simulink model "gm_Transformation_V12"  (R2022a)
settings: Solver=FixedStepDiscrete  StartTime=0.0  StopTime=10.0  RelTol=1e-3
InitFcn:
  | Ts_xadc = 0.1;
undefined symbols (not defined in the file or in its folder): T_25MHz, T_mech
libraries: hdlsllib x14, simulink x13, hdlmdlgenlib x6, simulink_need_slupdate x1
(part 1 of 4)
settings Model: Creator=trichte  LastModifiedBy=Andre Merx
settings SolverCC: AlgebraicLoopSolver=TrustRegion
settings DataIOCC: LimitDataPoints=on  SaveFormat=Array  SaveOutput=off  SaveTime=off  ReturnWorkspaceOutputs=off
settings OptimizationCC: BlockReduction=off  ConditionallyExecuteInputs=off  DefaultParameterBehavior=Inlined  LifeSpan=inf
settings DebuggingCC: AlgebraicLoopMsg=error  SolverPrmCheckMsg=warning  InheritedTsInSrcMsg=none  SingleTaskRateTransMsg=error  UnconnectedInputMsg=warning  UnconnectedOutputMsg=warning  UnconnectedLineMsg=warning  AllowSymbolicDim=off  StrictBusMsg=ErrorOnBusTreatedAsVector  SFUnexpectedBacktrackingDiag=warning  SFNoUnconditionalDefaultTransitionDiag=warning  SFExecutionAtInitializationDiag=none  SFMachineParentedDataDiag=warning  ArithmeticOperatorsInVariantConditions=warning
settings HardwareCC: ProdBitPerPointer=32  ProdBitPerSizeT=32  ProdBitPerPtrDiffT=32  ProdLargestAtomicFloat=None  ProdIntDivRoundTo=Undefined  ProdEndianess=Unspecified  ProdWordSize=32  ProdHWDeviceType=ASIC/FPGA->ASIC/FPGA  ProdEqTarget=off
settings ModelReferenceCC: PropagateSignalLabelsOutOfModel=off
settings SFSimCC: SimUseLocalCustomCode=off  CustomCodeUndefinedFunction=UseInterfaceOnly
settings RTWCC: RTWUseLocalCustomCode=off
settings CodeAppCC: StateflowObjectComments=on
settings GRTTargetCC: TargetLangStandard=C89/C90 (ANSI)
settings ConfigComp: CovMetricSettings=dw  CovSaveCumulativeToWorkspaceVar=on  CovSaveSingleToWorkspaceVar=on  CovExternalEMLEnable=off  CovSFcnEnable=off

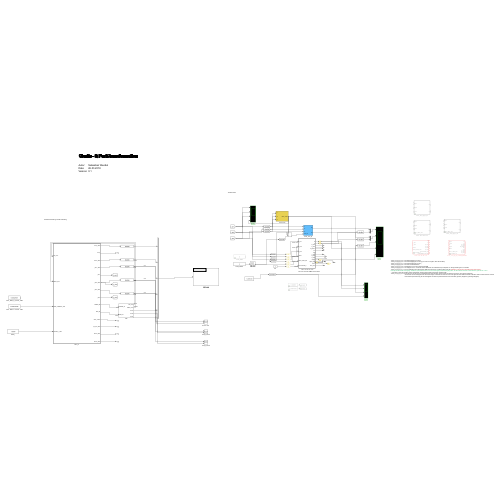
[thumbnail: Simulink's stored preview of the top-level diagram]
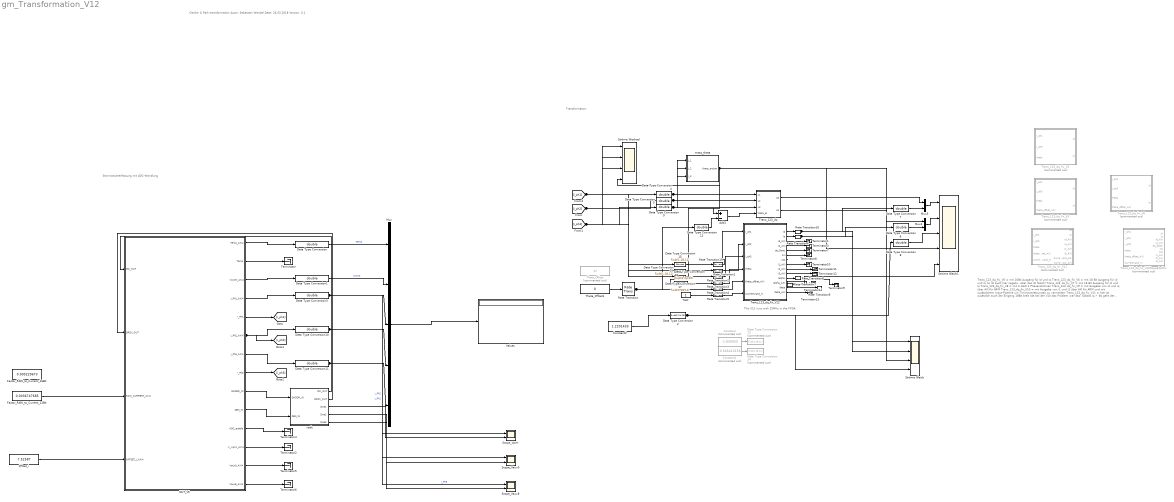
== system gm_Transformation_V12 ==
  note: Clarke- & Park-transformation
      |
      | Autor: Sebastian Wendel
      | Date: 26.03.2018
      | Version: 0.1
  note: Transformation
  note: Stromistwererfassung mit ADC-Wandlung
  note: Trans_123_dq_fix_V5 = mit 16Bit Ausgang für id und iq
      | Trans_123_dq_fix_V6 = mit 18 Bit Ausgang für id und iq (iq ist auch hier negativ, aber das ist falsch)
      | Trans_123_dq_fix_V7 = mit 18 Bit Ausgang für id und iq
      | Trans_123_dq_fix_V8 = mit 3 statt 2 Phasenströmen
      | Trans_123_dq_fix_V9 = mit Ausgabe von id und iq über AXI für ARM
      | Trans_123_dq_fix_V10 = mit Ausgabe von i1 und i3 über AXI für ARM und mit zusätzlichem Input-Pipeline um Timingverletzungen zu vermeiden
      | Trans_123_dq_fix_V11 = hier ist zusätzlich auch der Eingang 18Bit breit (da bei der V10 das Problem war das: Sobald iq > 9A geht der Trans-Block nicht mehr richtig...
      | Das liegt an den 16 Bit am Eingang. Sobald ich (wie bei den neunen V11 schon korregiert) 18 Bit am EIngang habe, ist das Problem behoben und der Bereich geht bis bis +/-36 A
      | ...ansonsten is alles wie gehabt. Wegen einheitlichen 18 Bit für alle Größem wird jedoch 18 Bit genutzt!
      | Trans_123_dq_fix_V12 = habe hier nun die dq-Trans von Saidi Said nicht mehr benutzt und bin auf die Verwendung von sinus und cosinus gewechselt.
      | da ich diese bei den VoltageVectors ohnehin benötige. Und hierdurch habe ich auch einen gleichen theta-offset für beide. Außerdem wollte ich alle 3 Ströme nehmen
      | Nach realer Implementierung ist die Genauigkeit von dieser dq-Transformation auch wesentlich genauer (doppelt so gute Bitgenauigkeit)
  note: This V12 runs with 25MHz in the FPGA.
  Add1 : Sum  Inputs=+-  OutDataTypeStr=Inherit: Same as accumulator
  Constant : Constant  Commented=on  Value=-1.839355
  Constant1 : Constant  Commented=on  Value=0.545410156
  Constant2 : Constant  Value=1.2201433
  DUT_V5 : Subsystem  TreatAsAtomicUnit=on
  Data Type Conversion{,1,3..12} (12 alike) : DataTypeConversion  OutDataTypeStr=double  SaturateOnIntegerOverflow=off  RndMeth=Floor
  Data Type Conversion13 : DataTypeConversion  Commented=on  OutDataTypeStr=fixdt(1,18,11)  SaturateOnIntegerOverflow=off  RndMeth=Floor
  Data Type Conversion14 : DataTypeConversion  Commented=on  OutDataTypeStr=fixdt(1,18,11)  SaturateOnIntegerOverflow=off  RndMeth=Floor
  Data Type Conversion15 : DataTypeConversion  OutDataTypeStr=fixdt(1,18,11)  SaturateOnIntegerOverflow=off  RndMeth=Floor
  Data Type Conversion16 : DataTypeConversion  OutDataTypeStr=fixdt(1,18,11)  SaturateOnIntegerOverflow=off  RndMeth=Floor
  Data Type Conversion17 : DataTypeConversion  OutDataTypeStr=fixdt(1,18,11)  SaturateOnIntegerOverflow=off  RndMeth=Floor
  Data Type Conversion18 : DataTypeConversion  OutDataTypeStr=fixdt(1,24,20)  SaturateOnIntegerOverflow=off  RndMeth=Floor
  Data Type Conversion2 : DataTypeConversion  OutDataTypeStr=fixdt(1,24,20)  SaturateOnIntegerOverflow=off  RndMeth=Floor
  Factor_RAW_to_Current_12Bit : Constant  Value=0.0036747685  OutDataTypeStr=fixdt(0,24,24)
  Factor_RAW_to_Current_16Bit : Constant  Value=0.000229673  OutDataTypeStr=fixdt(0,24,24)
  Mux : Mux  Inputs=5
  Mux3 : Mux  Inputs=2
  Mux4 : Mux  Inputs=2
  Offset_i : Constant  Value=7.52587  OutDataTypeStr=fixdt(0,16,11)
  Rate Transition{,6..9,16} (6 alike) : RateTransition  OutPortSampleTime=T_mech
  Rate Transition{1..5,19} (6 alike) : RateTransition  OutPortSampleTime=T_25MHz
  Scope_Vaux0 : Scope  NumInputPorts=2
  Scope_Vaux8 : Scope  NumInputPorts=2
  Scope_VpVn : Scope  NumInputPorts=2
  Ströme Gleich : Scope  NumInputPorts=4
  Ströme Gleich1 : Scope  NumInputPorts=5
  Ströme Wechsel : Scope  NumInputPorts=4
  Terminator{,1..14} (15 alike) : Terminator
  Test : Constant  OutDataTypeStr=boolean  SampleTime=T_mech
  Theta_Offset : Constant  Commented=on  Value=pi  OutDataTypeStr=fixdt(1,24,20)
  Theta_Offset1 : Constant  Value=0  OutDataTypeStr=fixdt(1,24,20)
  Trans_123_dq : Subsystem
  Trans_123_dq_fix_V11 : Subsystem  Commented=on  TreatAsAtomicUnit=on
  Trans_123_dq_fix_V12 : Subsystem  TreatAsAtomicUnit=on
  Trans_123_dq_fix_V12DoppelteMul : Subsystem  Commented=on  TreatAsAtomicUnit=on
  Trans_123_dq_fix_V3 : Subsystem  Commented=on  TreatAsAtomicUnit=on
  Trans_123_dq_fix_V5 : Subsystem  Commented=on  TreatAsAtomicUnit=on
  Trans_123_dq_fix_V6 : Subsystem  Commented=on  TreatAsAtomicUnit=on
  Values : Display
      settings: Format=hex (Stored Integer)
  meas_theta : Subsystem
  xadc : Subsystem
  wires:
  Trans_123_dq_fix_V12/12(ialpha_AXI) -> Terminator14/1
  Trans_123_dq_fix_V12/14(ibeta_AXI) -> Terminator13/1
  Trans_123_dq_fix_V12/13(ibeta) -> Rate Transition9/1
  Trans_123_dq_fix_V12/11(ialpha) -> Rate Transition8/1
  Rate Transition/1 -> Data Type Conversion12/1, Rate Transition4/1
  Data Type Conversion18/1 -> Rate Transition3/1
  Data Type Conversion17/1 -> Rate Transition2/1
  Data Type Conversion16/1 -> Rate Transition1/1
  Data Type Conversion15/1 -> Rate Transition19/1
  Trans_123_dq_fix_V12/7(cos) -> Rate Transition7/1
  Rate Transition6/1 -> Data Type Conversion6/1, Ströme Gleich/2
  Rate Transition16/1 -> Data Type Conversion7/1, Ströme Gleich/1
  Rate Transition5/1 -> Trans_123_dq_fix_V12/6(CurrentValid_in)
  Rate Transition4/1 -> Trans_123_dq_fix_V12/5(theta_offset_AXI)
  Rate Transition3/1 -> Trans_123_dq_fix_V12/4(theta)
  Rate Transition2/1 -> Trans_123_dq_fix_V12/3(i_ph3)
  Rate Transition1/1 -> Trans_123_dq_fix_V12/2(i_ph2)
  Rate Transition19/1 -> Trans_123_dq_fix_V12/1(i_ph1)
  Theta_Offset1/1 -> Rate Transition/1
  Trans_123_dq_fix_V12/10(i3_AXI) -> Terminator12/1
  Trans_123_dq_fix_V12/9(i2_AXI) -> Terminator11/1
  Constant2/1 -> Data Type Conversion2/1
  Constant1/1 -> Data Type Conversion14/1
  Constant/1 -> Data Type Conversion13/1
  Trans_123_dq_fix_V12/8(i1_AXI) -> Terminator10/1
  Test/1 -> Rate Transition5/1
  Rate Transition7/1 -> Terminator9/1, Ströme Gleich1/5
  [i_ph3] -> Data Type Conversion9/1, Data Type Conversion17/1, Ströme Wechsel/3
  [i_ph1] -> Data Type Conversion4/1, Data Type Conversion15/1, Ströme Wechsel/1
  Trans_123_dq_fix_V12/6(sin) -> Terminator8/1
  Trans_123_dq_fix_V12/5(dq_Done) -> Terminator7/1
  Trans_123_dq_fix_V12/3(id_AXI) -> Terminator1/1
  Trans_123_dq_fix_V12/4(iq_AXI) -> Terminator3/1
  Add1/1 -> Trans_123_dq/4(theta_el)
  Data Type Conversion12/1 -> Add1/2
  Trans_123_dq_fix_V12/2(iq) -> Rate Transition6/1
  Trans_123_dq_fix_V12/1(id) -> Rate Transition16/1
  [i_ph2] -> Data Type Conversion5/1, Data Type Conversion16/1, Ströme Wechsel/2
  DUT_V5/8(i_Ph3) -> [i_ph3]
  DUT_V5/5(i_Ph1) -> [i_ph1]
  Data Type Conversion5/1 -> Trans_123_dq/2(L2), meas_theta/2(I_2)
  Data Type Conversion9/1 -> Trans_123_dq/3(L3), meas_theta/3(I_3)
  Data Type Conversion4/1 -> Trans_123_dq/1(L1), meas_theta/1(I_1)
  meas_theta/1(theta_arctan) -> Add1/1, Data Type Conversion18/1, Ströme Gleich1/4, Ströme Gleich/3, Ströme Wechsel/4
  Data Type Conversion8/1 -> Ströme Gleich1/3
  Mux4/1 -> Ströme Gleich1/2
  Data Type Conversion6/1 -> Mux4/2
  Data Type Conversion7/1 -> Mux3/2
  Mux3/1 -> Ströme Gleich1/1
  Trans_123_dq/2(Uq) -> Mux4/1
  Trans_123_dq/1(Ud) -> Mux3/1
  Data Type Conversion2/1 -> Data Type Conversion8/1, Ströme Gleich/4
  xadc/5(Sine3) -> Scope_Vaux8/2
  xadc/4(Sine2) -> Scope_Vaux0/2
  xadc/3(Sine1) -> Scope_VpVn/2
  DUT_V5/14(Vaux8_AXI4) -> Terminator6/1
  DUT_V5/13(Vaux0_AXI4) -> Terminator5/1
  DUT_V5/12(V_VpVn_AXI4) -> Terminator2/1
  Offset_i/1 -> DUT_V5/4(OFFSET_I_AXI4)
  Factor_RAW_to_Current_12Bit/1 -> DUT_V5/3(RAW_CURRENT_AXI4)
  DUT_V5/11(ADC_enable) -> Terminator4/1
  DUT_V5/2(Temp) -> Terminator/1
  xadc/1(DO_OUT) -> DUT_V5/1(DO_OUT)
  xadc/2(DRDY_OUT) -> DUT_V5/2(DRDY_OUT)
  DUT_V5/10(DEN_IN) -> xadc/2(DEN_IN)
  DUT_V5/9(DADDR_IN) -> xadc/1(DADDR_IN)
  Data Type Conversion1/1 -> Mux/2  "VccInt"
  Data Type Conversion11/1 -> Mux/5, Scope_Vaux8/1  "i_Ph3"
  Data Type Conversion10/1 -> Mux/4, Scope_Vaux0/1  "i_Ph2"
  Data Type Conversion3/1 -> Mux/3, Scope_VpVn/1  "i_Ph1"
  Data Type Conversion/1 -> Mux/1  "Temp"
  Mux/1 -> Values/1
  DUT_V5/6(i_Ph2_AXI4) -> Data Type Conversion10/1, [i_ph2]
  DUT_V5/7(i_Ph3_AXI4) -> Data Type Conversion11/1
  DUT_V5/4(i_Ph1_AXI4) -> Data Type Conversion3/1
  DUT_V5/3(VccInt_AXI4) -> Data Type Conversion1/1
  DUT_V5/1(Temp_AXI4) -> Data Type Conversion/1

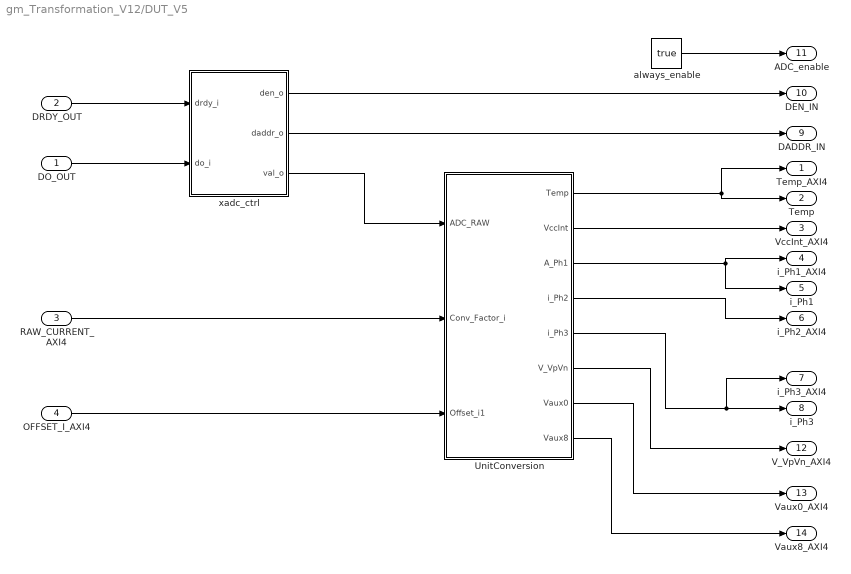
== system gm_Transformation_V12/DUT_V5 ==
  DO_OUT : Inport
  DRDY_OUT : Inport  Port=2
  RAW_CURRENT_AXI4 : Inport  Port=3
  OFFSET_I_AXI4 : Inport  Port=4
  UnitConversion : Subsystem
  always_enable : Constant  Value=true  OutDataTypeStr=boolean
  xadc_ctrl : MATLAB Function  TreatAsAtomicUnit=on
  Temp_AXI4 : Outport  VectorParamsAs1DForOutWhenUnconnected=off
  Temp : Outport  Port=2  VectorParamsAs1DForOutWhenUnconnected=off
  VccInt_AXI4 : Outport  Port=3  VectorParamsAs1DForOutWhenUnconnected=off
  i_Ph1_AXI4 : Outport  Port=4  VectorParamsAs1DForOutWhenUnconnected=off
  i_Ph1 : Outport  Port=5  VectorParamsAs1DForOutWhenUnconnected=off
  i_Ph2_AXI4 : Outport  Port=6  VectorParamsAs1DForOutWhenUnconnected=off
  i_Ph3_AXI4 : Outport  Port=7  VectorParamsAs1DForOutWhenUnconnected=off
  i_Ph3 : Outport  Port=8  VectorParamsAs1DForOutWhenUnconnected=off
  DADDR_IN : Outport  Port=9  VectorParamsAs1DForOutWhenUnconnected=off
  DEN_IN : Outport  Port=10  VectorParamsAs1DForOutWhenUnconnected=off
  ADC_enable : Outport  Port=11  VectorParamsAs1DForOutWhenUnconnected=off
  V_VpVn_AXI4 : Outport  Port=12  VectorParamsAs1DForOutWhenUnconnected=off
  Vaux0_AXI4 : Outport  Port=13  VectorParamsAs1DForOutWhenUnconnected=off
  Vaux8_AXI4 : Outport  Port=14  VectorParamsAs1DForOutWhenUnconnected=off
  wires:
  UnitConversion/8(Vaux8) -> Vaux8_AXI4/1
  UnitConversion/7(Vaux0) -> Vaux0_AXI4/1
  OFFSET_I_AXI4/1 -> UnitConversion/3(Offset_i1)
  UnitConversion/6(V_VpVn) -> V_VpVn_AXI4/1
  RAW_CURRENT_AXI4/1 -> UnitConversion/2(Conv_Factor_i)
  always_enable/1 -> ADC_enable/1
  xadc_ctrl/2(daddr_o) -> DADDR_IN/1
  xadc_ctrl/1(den_o) -> DEN_IN/1
  DO_OUT/1 -> xadc_ctrl/2(do_i)
  DRDY_OUT/1 -> xadc_ctrl/1(drdy_i)
  UnitConversion/1(Temp) -> Temp_AXI4/1, Temp/1
  UnitConversion/2(VccInt) -> VccInt_AXI4/1
  UnitConversion/4(i_Ph2) -> i_Ph2_AXI4/1
  UnitConversion/3(A_Ph1) -> i_Ph1_AXI4/1, i_Ph1/1
  UnitConversion/5(i_Ph3) -> i_Ph3_AXI4/1, i_Ph3/1
  xadc_ctrl/3(val_o) -> UnitConversion/1(ADC_RAW)

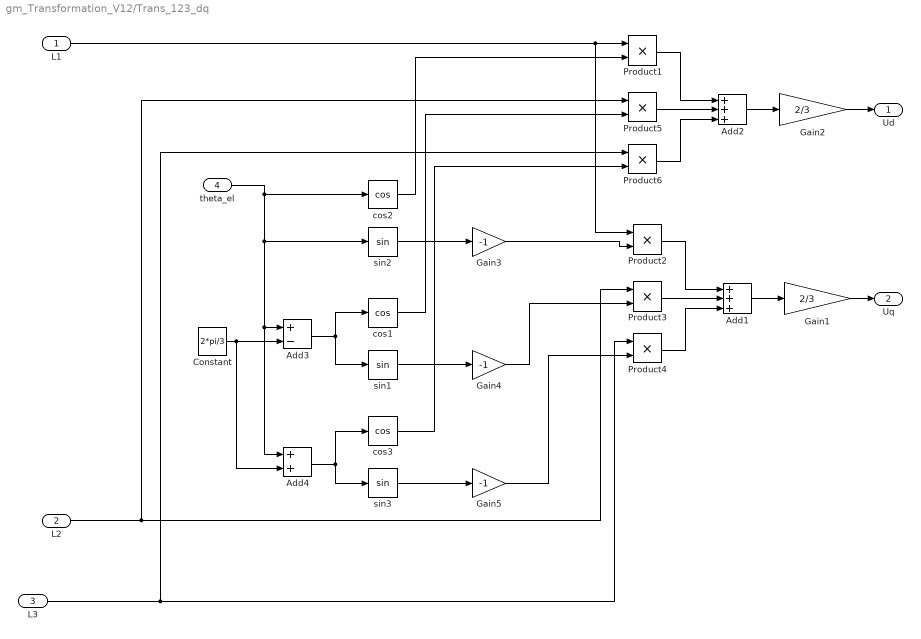
== system gm_Transformation_V12/Trans_123_dq ==
  L1 : Inport
  L2 : Inport  Port=2
  L3 : Inport  Port=3
  theta_el : Inport  Port=4
  Add1 : Sum  Inputs=+++
  Add2 : Sum  Inputs=+++
  Add3 : Sum  Inputs=+-
  Add4 : Sum
  Constant : Constant  Value=2*pi/3  SampleTime=T_mech
  Gain1 : Gain  Gain=2/3
  Gain2 : Gain  Gain=2/3
  Gain3 : Gain  Gain=-1
  Gain4 : Gain  Gain=-1
  Gain5 : Gain  Gain=-1
  Product{1..6} (6 alike) : Product  RndMeth=Zero
  cos1 : Trigonometry  Operator=cos
  cos2 : Trigonometry  Operator=cos
  cos3 : Trigonometry  Operator=cos
  sin1 : Trigonometry
  sin2 : Trigonometry
  sin3 : Trigonometry
  Ud : Outport  VectorParamsAs1DForOutWhenUnconnected=off
  Uq : Outport  Port=2  VectorParamsAs1DForOutWhenUnconnected=off
  wires:
  cos2/1 -> Product1/2
  cos1/1 -> Product5/2
  cos3/1 -> Product6/2
  Product1/1 -> Add2/1
  Add4/1 -> sin3/1, cos3/1
  Add3/1 -> sin1/1, cos1/1
  Constant/1 -> Add4/2, Add3/2
  theta_el/1 -> sin2/1, Add4/1, Add3/1, cos2/1
  Product3/1 -> Add1/2
  Product2/1 -> Add1/1
  Add1/1 -> Gain1/1
  Product4/1 -> Add1/3
  Product5/1 -> Add2/2
  Add2/1 -> Gain2/1
  Product6/1 -> Add2/3
  Gain2/1 -> Ud/1
  Gain1/1 -> Uq/1
  L1/1 -> Product1/1, Product2/1
  L2/1 -> Product5/1, Product3/1
  L3/1 -> Product6/1, Product4/1
  sin2/1 -> Gain3/1
  sin1/1 -> Gain4/1
  sin3/1 -> Gain5/1
  Gain3/1 -> Product2/2
  Gain4/1 -> Product3/2
  Gain5/1 -> Product4/2

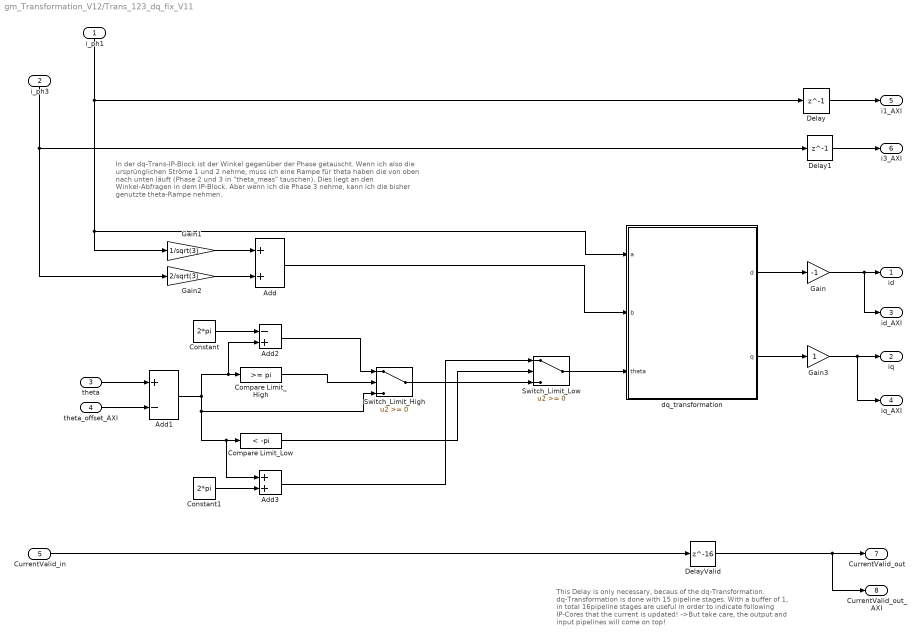
== system gm_Transformation_V12/Trans_123_dq_fix_V11 ==
  note: In der dq-Trans-IP-Block ist der Winkel gegenüber der Phase getauscht.
      | Wenn ich also die ursprünglichen Ströme 1 und 2 nehme,
      |  muss ich eine Rampe für theta haben die von oben nach unten läuft
      | (Phase 2 und 3 in "theta_meas" tauschen).
      | Dies liegt an den Winkel-Abfragen in dem IP-Block.
      | Aber wenn ich die Phase 3 nehme, kann ich die bisher genutzte theta-Rampe nehmen.
  note: This Delay is only necessary, becaus of the dq-Transformation.
      | dq-Transformation is done with 15 pipeline stages.
      | With a buffer of 1, in total 16pipeline stages are useful in order to
      |  indicate following IP-Cores that the current is updated!
      | ->But take care, the output and input pipelines will come on top!
  i_ph1 : Inport
  i_ph3 : Inport  Port=2
  theta : Inport  Port=3
  theta_offset_AXI : Inport  Port=4
  CurrentValid_in : Inport  Port=5
  Add : Sum
  Add1 : Sum  Inputs=+-  OutDataTypeStr=Inherit: Same as accumulator
  Add2 : Sum  Inputs=-+  OutDataTypeStr=Inherit: Same as first input
  Add3 : Sum  OutDataTypeStr=Inherit: Same as first input
  Compare Limit_High : simulink/Logic and Bit Operations/Compare To Constant  relop=>=  const=pi  OutDataTypeStr=boolean
  Compare Limit_Low : simulink/Logic and Bit Operations/Compare To Constant  relop=<  const=-pi  OutDataTypeStr=boolean
  Constant : Constant  Value=2*pi  OutDataTypeStr=fixdt(1,24,20)  SampleTime=-1
  Constant1 : Constant  Value=2*pi  OutDataTypeStr=fixdt(1,24,20)  SampleTime=-1
  Delay : Delay  DelayLength=1
  Delay1 : Delay  DelayLength=1
  DelayValid : Delay  DelayLength=16
  Gain : Gain  Gain=-1  OutDataTypeStr=fixdt(1,18,11)
  Gain1 : Gain  Gain=1/sqrt(3)  OutDataTypeStr=Inherit: Same as input
  Gain2 : Gain  Gain=2/sqrt(3)  OutDataTypeStr=Inherit: Same as input
  Gain3 : Gain  OutDataTypeStr=fixdt(1,18,11)
  Switch_Limit_High : Switch  OutDataTypeStr=fixdt(1,24,20)  SaturateOnIntegerOverflow=off  InputSameDT=off
  Switch_Limit_Low : Switch  OutDataTypeStr=fixdt(1,24,20)  SaturateOnIntegerOverflow=off  InputSameDT=off
  dq_transformation : MATLAB Function  TreatAsAtomicUnit=on
  id : Outport  VectorParamsAs1DForOutWhenUnconnected=off
  iq : Outport  Port=2  VectorParamsAs1DForOutWhenUnconnected=off
  id_AXI : Outport  Port=3  VectorParamsAs1DForOutWhenUnconnected=off
  iq_AXI : Outport  Port=4  VectorParamsAs1DForOutWhenUnconnected=off
  i1_AXI : Outport  Port=5  VectorParamsAs1DForOutWhenUnconnected=off
  i3_AXI : Outport  Port=6  VectorParamsAs1DForOutWhenUnconnected=off
  CurrentValid_out : Outport  Port=7  VectorParamsAs1DForOutWhenUnconnected=off
  CurrentValid_out_AXI : Outport  Port=8  VectorParamsAs1DForOutWhenUnconnected=off
  wires:
  CurrentValid_in/1 -> DelayValid/1
  DelayValid/1 -> CurrentValid_out/1, CurrentValid_out_AXI/1
  i_ph1/1 -> Delay/1, dq_transformation/1(a), Gain1/1
  i_ph3/1 -> Delay1/1, Gain2/1
  Delay1/1 -> i3_AXI/1
  Delay/1 -> i1_AXI/1
  Gain/1 -> id/1, id_AXI/1
  Gain3/1 -> iq/1, iq_AXI/1
  Add3/1 -> Switch_Limit_Low/1
  Constant1/1 -> Add3/2
  Add2/1 -> Switch_Limit_High/1
  Constant/1 -> Add2/1
  Compare Limit_Low/1 -> Switch_Limit_Low/2
  Compare Limit_High/1 -> Switch_Limit_High/2
  Switch_Limit_High/1 -> Switch_Limit_Low/3
  Switch_Limit_Low/1 -> dq_transformation/3(theta)
  theta_offset_AXI/1 -> Add1/2
  Add1/1 -> Compare Limit_High/1, Add2/2, Compare Limit_Low/1, Add3/1, Switch_Limit_High/3
  theta/1 -> Add1/1
  dq_transformation/1(d) -> Gain/1
  dq_transformation/2(q) -> Gain3/1
  Gain2/1 -> Add/2
  Gain1/1 -> Add/1
  Add/1 -> dq_transformation/2(b)

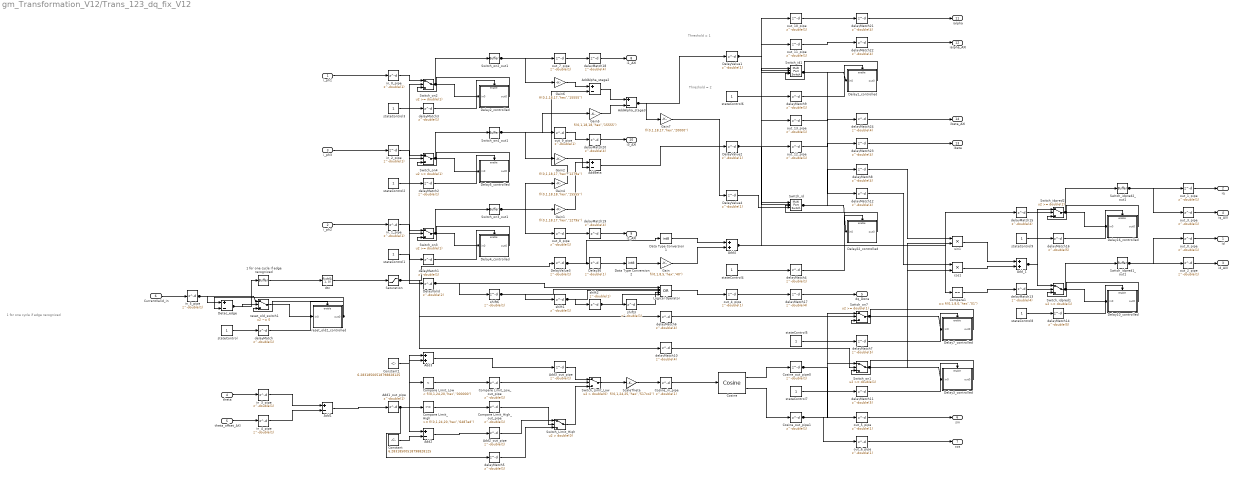
== system gm_Transformation_V12/Trans_123_dq_fix_V12 ==
  note: Threshold = 2
  note: Threshold = 1
  note: 1 for one cycle if edge recognized
  i_ph1 : Inport  OutDataTypeStr=fixdt(1, 18, 11)  PortDimensions=1  SampleTime=4e-08
  i_ph2 : Inport  Port=2  OutDataTypeStr=fixdt(1, 18, 11)  PortDimensions=1  SampleTime=4e-08
  i_ph3 : Inport  Port=3  OutDataTypeStr=fixdt(1, 18, 11)  PortDimensions=1  SampleTime=4e-08
  theta : Inport  Port=4  OutDataTypeStr=fixdt(1, 24, 20)  PortDimensions=1  SampleTime=4e-08
  theta_offset_AXI : Inport  Port=5  OutDataTypeStr=fixdt(1, 24, 20)  PortDimensions=1  SampleTime=4e-08
  CurrentValid_in : Inport  Port=6  OutDataTypeStr=boolean  PortDimensions=1  SampleTime=4e-08
  1 for one cycle if edge recognized : hdlmdlgenlib/Buffer
      settings: SourceProductBaseCode=SL
  Add1 : Sum  Inputs=+-  AccumDataTypeStr=fixdt(1, 24, 20)  OutDataTypeStr=fixdt(1, 24, 20)  SampleTime=4e-08
  Add1_out_pipe : Delay  DelayLength=double(1)  InitialCondition=0  SampleTime=4e-08
  Add2 : Sum  Inputs=+-  AccumDataTypeStr=fixdt(1, 24, 20)  OutDataTypeStr=fixdt(1, 24, 20)  SampleTime=4e-08
  Add2_out_pipe : Delay  DelayLength=double(1)  InitialCondition=0  SampleTime=4e-08
  Add3 : Sum  AccumDataTypeStr=fixdt(1, 24, 20)  OutDataTypeStr=fixdt(1, 24, 20)  SampleTime=4e-08
  Add3_out_pipe : Delay  DelayLength=double(1)  InitialCondition=0  SampleTime=4e-08
  Add4 : Sum  AccumDataTypeStr=int8  OutDataTypeStr=int8  RndMeth=Simplest  SampleTime=4e-08
  AddAlpha_stage2 : Sum  Inputs=+-  AccumDataTypeStr=fixdt(1, 18, 11)  OutDataTypeStr=fixdt(1, 18, 11)  SampleTime=4e-08
  AddAlpha_stage3 : Sum  Inputs=+-  AccumDataTypeStr=fixdt(1, 18, 11)  OutDataTypeStr=fixdt(1, 18, 11)  SampleTime=4e-08
  AddBeta : Sum  Inputs=+-  AccumDataTypeStr=fixdt(1, 18, 11)  OutDataTypeStr=fixdt(1, 18, 11)  SampleTime=4e-08
  Add_1 : Sum  AccumDataTypeStr=fixdt(1, 18, 11)  OutDataTypeStr=fixdt(1, 18, 11)  SampleTime=4e-08
  Compare Limit_High : simulink/Logic and Bit Operations/Compare To Constant  relop=>=  const="fi(0,1,24,20,\"hex\",\"6487ed\")"  OutDataTypeStr=boolean
  Compare Limit_High_out_pipe : Delay  DelayLength=double(1)  InitialCondition=0  SampleTime=4e-08
  Compare Limit_Low : simulink/Logic and Bit Operations/Compare To Constant  relop=<  const="fi(0,1,24,20,\"hex\",\"000000\")"  OutDataTypeStr=boolean
  Compare Limit_Low_out_pipe : Delay  DelayLength=double(1)  InitialCondition=0  SampleTime=4e-08
  Compare1 : simulink/Logic and Bit Operations/Compare To Constant  relop===  const="fi(0,1,8,0,\"hex\",\"01\")"  OutDataTypeStr=boolean
  Constant : Constant  Value=6.28318500518798828125  OutDataTypeStr=fixdt(1, 24, 20)  SampleTime=4e-08
  Constant1 : Constant  Value=6.28318500518798828125  OutDataTypeStr=fixdt(1, 24, 20)  SampleTime=4e-08
  Cosine : simulink/Lookup Tables/Cosine  Formula=sin(2*pi*u) and cos(2*pi*u)  NumDataPoints=(2^9)+1  OutputWordLength=16  InternalRulePriority=Precision
      settings: SourceProductBaseCode=SL
  Cosine_in_pipe : Delay  DelayLength=double(1)  InitialCondition=0  SampleTime=4e-08
  Cosine_out_pipe0 : Delay  DelayLength=double(1)  InitialCondition=0  SampleTime=4e-08
  Cosine_out_pipe1 : Delay  DelayLength=double(1)  InitialCondition=0  SampleTime=4e-08
  Data Type Conversion1 : DataTypeConversion  OutDataTypeStr=int8  SampleTime=4e-08  SaturateOnIntegerOverflow=off  RndMeth=Floor
  Data Type Conversion2 : DataTypeConversion  OutDataTypeStr=int8  SampleTime=4e-08  SaturateOnIntegerOverflow=off  RndMeth=Floor
  Delay10_controlled : Subsystem
  Delay16_controlled : Subsystem
  Delay1_controlled : Subsystem
  Delay22_controlled : Subsystem
  Delay2_controlled : Subsystem
  Delay36 : Delay  DelayLength=double(1)  InitialCondition=0  SampleTime=4e-08
  Delay3_controlled : Subsystem
  Delay4_controlled : Subsystem
  Delay5_controlled : Subsystem
  Delay7_controlled : Subsystem
  DelayValid : Delay  DelayLength=double(2)  InitialCondition=0  SampleTime=4e-08
  DelayValue{1..4} (4 alike) : Delay  DelayLength=double(1)  InitialCondition=0  SampleTime=4e-08
  Detec_edge : Sum  Inputs=+-  AccumDataTypeStr=int8  OutDataTypeStr=int8  SampleTime=4e-08
  Gain : Gain  Gain="fi(0,1,8,5,\"hex\",\"40\")"  ParamDataTypeStr=fixdt(1, 8, 5)  OutDataTypeStr=fixdt(1, 16, 5)  RndMeth=Simplest  SampleTime=4e-08
  Gain1 : Gain  Gain="fi(0,1,18,17,\"hex\",\"1279a\")"  ParamDataTypeStr=fixdt(1, 18, 17)  OutDataTypeStr=fixdt(1, 18, 11)  SampleTime=4e-08
  Gain2 : Gain  Gain="fi(0,1,18,17,\"hex\",\"1279a\")"  ParamDataTypeStr=fixdt(1, 18, 17)  OutDataTypeStr=fixdt(1, 18, 11)  SampleTime=4e-08
  Gain4 : Gain  Gain="fi(0,1,18,18,\"hex\",\"15555\")"  ParamDataTypeStr=fixdt(1, 18, 18)  OutDataTypeStr=fixdt(1, 18, 11)  SampleTime=4e-08
  Gain5 : Gain  Gain="fi(0,1,18,18,\"hex\",\"15555\")"  ParamDataTypeStr=fixdt(1, 18, 18)  OutDataTypeStr=fixdt(1, 18, 11)  SampleTime=4e-08
  Gain6 : Gain  Gain="fi(0,1,18,17,\"hex\",\"15555\")"  ParamDataTypeStr=fixdt(1, 18, 17)  OutDataTypeStr=fixdt(1, 18, 11)  SampleTime=4e-08
  Gain7 : Gain  Gain="fi(0,1,18,17,\"hex\",\"20000\")"  ParamDataTypeStr=fixdt(1, 18, 17)  OutDataTypeStr=fixdt(1, 18, 11)  SampleTime=4e-08
  Logical Operator : Logic  Operator=OR  Inputs=5  AllPortsSameDT=off  OutDataTypeStr=boolean  SampleTime=4e-08
  Saturation : Saturate  UpperLimit="fi(0,0,1,0,\"hex\",\"1\")"  LowerLimit="fi(0,0,1,0,\"hex\",\"0\")"  SampleTime=4e-08  OutDataTypeStr=fixdt(0, 1, 0)
  ScaleTheta : Gain  Gain="fi(0,1,24,25,\"hex\",\"517cc2\")"  ParamDataTypeStr=fixdt(1, 24, 25)  OutDataTypeStr=fixdt(1, 24, 20)  SampleTime=4e-08
  Switch_Limit_High : Switch  Criteria=u2 > Threshold  Threshold=double(0)  OutDataTypeStr=fixdt(1, 24, 20)  SampleTime=4e-08  SaturateOnIntegerOverflow=off  InputSameDT=off
  Switch_Limit_Low : Switch  Criteria=u2 > Threshold  Threshold=double(0)  OutDataTypeStr=fixdt(1, 24, 20)  SampleTime=4e-08  SaturateOnIntegerOverflow=off  InputSameDT=off
  Switch_id : MultiPortSwitch  Inputs=2  DataPortForDefault=Additional data port  DiagnosticForDefault=None  OutDataTypeStr=fixdt(1, 18, 11)  RndMeth=Simplest  SampleTime=4e-08  SaturateOnIntegerOverflow=off  InputSameDT=off
  Switch_id1 : MultiPortSwitch  Inputs=2  DataPortForDefault=Additional data port  DiagnosticForDefault=None  OutDataTypeStr=fixdt(1, 18, 11)  RndMeth=Simplest  SampleTime=4e-08  SaturateOnIntegerOverflow=off  InputSameDT=off
  Switch_idpred1 : Switch  Threshold=double(1)  OutDataTypeStr=fixdt(1, 18, 11)  RndMeth=Simplest  SampleTime=4e-08  SaturateOnIntegerOverflow=off  InputSameDT=off
  Switch_idpred1_out1 : hdlmdlgenlib/Buffer
      settings: SourceProductBaseCode=SL
  Switch_idpred2 : Switch  Threshold=double(2)  OutDataTypeStr=fixdt(1, 18, 11)  RndMeth=Simplest  SampleTime=4e-08  SaturateOnIntegerOverflow=off  InputSameDT=off
  Switch_idpred2_out1 : hdlmdlgenlib/Buffer
      settings: SourceProductBaseCode=SL
  Switch_on1 : Switch  Threshold=double(1)  OutDataTypeStr=fixdt(1, 16, 14)  SampleTime=4e-08  SaturateOnIntegerOverflow=off  InputSameDT=off
  Switch_on2 : Switch  Threshold=double(1)  OutDataTypeStr=fixdt(1, 18, 11)  RndMeth=Simplest  SampleTime=4e-08  SaturateOnIntegerOverflow=off  InputSameDT=off
  Switch_on2_out1 : hdlmdlgenlib/Buffer
      settings: SourceProductBaseCode=SL
  Switch_on3 : Switch  Threshold=double(1)  OutDataTypeStr=fixdt(1, 18, 11)  RndMeth=Simplest  SampleTime=4e-08  SaturateOnIntegerOverflow=off  InputSameDT=off
  Switch_on3_out1 : hdlmdlgenlib/Buffer
      settings: SourceProductBaseCode=SL
  Switch_on4 : Switch  Threshold=double(1)  OutDataTypeStr=fixdt(1, 18, 11)  RndMeth=Simplest  SampleTime=4e-08  SaturateOnIntegerOverflow=off  InputSameDT=off
  Switch_on4_out1 : hdlmdlgenlib/Buffer
      settings: SourceProductBaseCode=SL
  Switch_on7 : Switch  Threshold=double(1)  OutDataTypeStr=fixdt(1, 16, 14)  SampleTime=4e-08  SaturateOnIntegerOverflow=off  InputSameDT=off
  cos1 : Product  Inputs=**  OutDataTypeStr=fixdt(1, 18, 11)  RndMeth=Simplest  SampleTime=4e-08
  delayMatch{,1..5,9} (7 alike) : Delay  DelayLength=double(1)  InitialCondition=0  SampleTime=4e-08
  delayMatch{6,8,10,12..13,15,17..24} (14 alike) : Delay  DelayLength=double(4)  InitialCondition=0  SampleTime=4e-08
  delayMatch{7,11,14,16} (4 alike) : Delay  DelayLength=double(5)  InitialCondition=0  SampleTime=4e-08
  dtc : DataTypeConversion  OutDataTypeStr=fixdt(0, 1, 0)  SampleTime=4e-08  RndMeth=Floor
  in_0_pipe : Delay  DelayLength=double(1)  InitialCondition=0  SampleTime=4e-08
  in_1_pipe : Delay  DelayLength=double(1)  InitialCondition=0  SampleTime=4e-08
  in_2_pipe : Delay  DelayLength=double(1)  InitialCondition=0  SampleTime=4e-08
  in_3_pipe : Delay  DelayLength=double(1)  InitialCondition=0  SampleTime=4e-08
  in_4_pipe : Delay  DelayLength=double(1)  InitialCondition=0  SampleTime=4e-08
  in_5_pipe : Delay  DelayLength=double(1)  InitialCondition=0  SampleTime=4e-08
  out_0_pipe : Delay  DelayLength=double(1)  InitialCondition=0  SampleTime=4e-08
  out_10_pipe : Delay  DelayLength=double(1)  InitialCondition=0  SampleTime=4e-08
  out_11_pipe : Delay  DelayLength=double(1)  InitialCondition=0  SampleTime=4e-08
  out_12_pipe : Delay  DelayLength=double(1)  InitialCondition=0  SampleTime=4e-08
  out_13_pipe : Delay  DelayLength=double(1)  InitialCondition=0  SampleTime=4e-08
  out_1_pipe : Delay  DelayLength=double(1)  InitialCondition=0  SampleTime=4e-08
  out_2_pipe : Delay  DelayLength=double(1)  InitialCondition=0  SampleTime=4e-08
  out_3_pipe : Delay  DelayLength=double(1)  InitialCondition=0  SampleTime=4e-08
  out_4_pipe : Delay  DelayLength=double(1)  InitialCondition=0  SampleTime=4e-08
  out_5_pipe : Delay  DelayLength=double(1)  InitialCondition=0  SampleTime=4e-08
  out_6_pipe : Delay  DelayLength=double(1)  InitialCondition=0  SampleTime=4e-08
  out_7_pipe : Delay  DelayLength=double(1)  InitialCondition=0  SampleTime=4e-08
  out_8_pipe : Delay  DelayLength=double(1)  InitialCondition=0  SampleTime=4e-08
  out_9_pipe : Delay  DelayLength=double(1)  InitialCondition=0  SampleTime=4e-08
  reset_old2_controlled : Subsystem
  reset_old_switch1 : Switch  Criteria=u2 ~= 0  Threshold=double(0)  OutDataTypeStr=boolean  SampleTime=4e-08  SaturateOnIntegerOverflow=off  InputSameDT=off
  shift{1..3,6} (4 alike) : Delay  DelayLength=double(1)  InitialCondition=0  SampleTime=4e-08
  sin1 : Product  Inputs=**  OutDataTypeStr=fixdt(1, 18, 11)  RndMeth=Simplest  SampleTime=4e-08
  stateControl{,1..9} (10 alike) : Constant  OutDataTypeStr=boolean  SampleTime=4e-08
  id : Outport  SampleTime=4e-08  VectorParamsAs1DForOutWhenUnconnected=off
  iq : Outport  Port=2  SampleTime=4e-08  VectorParamsAs1DForOutWhenUnconnected=off
  id_AXI : Outport  Port=3  SampleTime=4e-08  VectorParamsAs1DForOutWhenUnconnected=off
  iq_AXI : Outport  Port=4  SampleTime=4e-08  VectorParamsAs1DForOutWhenUnconnected=off
  dq_Done : Outport  Port=5  SampleTime=4e-08  VectorParamsAs1DForOutWhenUnconnected=off
  sin : Outport  Port=6  SampleTime=4e-08  VectorParamsAs1DForOutWhenUnconnected=off
  cos : Outport  Port=7  SampleTime=4e-08  VectorParamsAs1DForOutWhenUnconnected=off
  i1_AXI : Outport  Port=8  SampleTime=4e-08  VectorParamsAs1DForOutWhenUnconnected=off
  i2_AXI : Outport  Port=9  SampleTime=4e-08  VectorParamsAs1DForOutWhenUnconnected=off
  i3_AXI : Outport  Port=10  SampleTime=4e-08  VectorParamsAs1DForOutWhenUnconnected=off
  ialpha : Outport  Port=11  SampleTime=4e-08  VectorParamsAs1DForOutWhenUnconnected=off
  ialpha_AXI : Outport  Port=12  SampleTime=4e-08  VectorParamsAs1DForOutWhenUnconnected=off
  ibeta : Outport  Port=13  SampleTime=4e-08  VectorParamsAs1DForOutWhenUnconnected=off
  ibeta_AXI : Outport  Port=14  SampleTime=4e-08  VectorParamsAs1DForOutWhenUnconnected=off
  wires:
  in_0_pipe/1 -> Switch_on2/1
  in_1_pipe/1 -> Switch_on3/1
  in_2_pipe/1 -> Switch_on4/1
  in_3_pipe/1 -> Add1/1
  in_4_pipe/1 -> Add1/2
  in_5_pipe/1 -> reset_old_switch1/1, Detec_edge/1
  delayMatch5/1 -> Switch_Limit_High/3
  Add2_out_pipe/1 -> Switch_Limit_High/1
  Add3_out_pipe/1 -> Switch_Limit_Low/1
  delayMatch15/1 -> Switch_idpred2/2
  AddAlpha_stage3/1 -> Gain7/1, DelayValue1/1
  AddBeta/1 -> DelayValue2/1
  Add_1/1 -> Switch_idpred1/1, Switch_idpred2/1
  Compare Limit_High_out_pipe/1 -> Switch_Limit_High/2
  Compare Limit_Low_out_pipe/1 -> Switch_Limit_Low/2
  delayMatch13/1 -> Switch_idpred1/2
  Constant/1 -> Add2/2
  Constant1/1 -> Add3/2
  Cosine_out_pipe0/1 -> out_5_pipe/1, Switch_on7/1
  Cosine_out_pipe1/1 -> out_6_pipe/1, Switch_on1/1
  Data Type Conversion1/1 -> Add4/1
  Data Type Conversion2/1 -> Gain/1
  Delay36/1 -> Data Type Conversion2/1
  DelayValid/1 -> Logical Operator/1, shift6/1
  DelayValue1/1 -> out_11_pipe/1, out_10_pipe/1, Switch_id1/2
  DelayValue2/1 -> out_13_pipe/1, out_12_pipe/1, Switch_id/2, Switch_id1/3
  DelayValue3/1 -> Data Type Conversion1/1, Delay36/1
  DelayValue4/1 -> Switch_id/3
  1 for one cycle if edge recognized/1 -> dtc/1
  Gain/1 -> Add4/2
  Gain1/1 -> AddBeta/1
  Gain2/1 -> AddBeta/2
  Gain4/1 -> AddAlpha_stage2/2
  Gain5/1 -> AddAlpha_stage3/2
  Gain6/1 -> AddAlpha_stage2/1
  Gain7/1 -> DelayValue4/1
  Logical Operator/1 -> out_4_pipe/1
  delayMatch6/1 -> Switch_on7/2
  ScaleTheta/1 -> Cosine_in_pipe/1
  Switch_Limit_High/1 -> Switch_Limit_Low/3
  Switch_Limit_Low/1 -> ScaleTheta/1
  delayMatch8/1 -> sin1/1
  delayMatch12/1 -> cos1/1
  Switch_idpred1_out1/1 -> out_2_pipe/1, out_0_pipe/1
  Switch_idpred2_out1/1 -> out_3_pipe/1, out_1_pipe/1
  Switch_on2_out1/1 -> out_7_pipe/1, Gain6/1
  Switch_on3_out1/1 -> out_8_pipe/1, Gain4/1, Gain1/1
  Switch_on4_out1/1 -> out_9_pipe/1, Gain5/1, Gain2/1
  cos1/1 -> Add_1/2
  shift1/1 -> Logical Operator/3, shift2/1
  shift2/1 -> Logical Operator/4, shift3/1
  shift3/1 -> Logical Operator/5
  shift6/1 -> Logical Operator/2, shift1/1
  sin1/1 -> Add_1/1
  out_0_pipe/1 -> id/1
  out_1_pipe/1 -> iq/1
  out_2_pipe/1 -> id_AXI/1
  out_3_pipe/1 -> iq_AXI/1
  delayMatch17/1 -> dq_Done/1
  out_5_pipe/1 -> sin/1
  out_6_pipe/1 -> cos/1
  delayMatch18/1 -> i1_AXI/1
  delayMatch19/1 -> i2_AXI/1
  delayMatch20/1 -> i3_AXI/1
  delayMatch21/1 -> ialpha/1
  delayMatch22/1 -> ialpha_AXI/1
  delayMatch23/1 -> ibeta/1
  delayMatch24/1 -> ibeta_AXI/1
  Add1/1 -> Add1_out_pipe/1
  Add2/1 -> Add2_out_pipe/1
  Add3/1 -> Add3_out_pipe/1
  Compare Limit_High/1 -> Compare Limit_High_out_pipe/1
  Compare Limit_Low/1 -> Compare Limit_Low_out_pipe/1
  i_ph1/1 -> in_0_pipe/1
  i_ph2/1 -> in_1_pipe/1
  i_ph3/1 -> in_2_pipe/1
  theta/1 -> in_3_pipe/1
  theta_offset_AXI/1 -> in_4_pipe/1
  CurrentValid_in/1 -> in_5_pipe/1
  Cosine/1 -> Cosine_out_pipe0/1
  Cosine/2 -> Cosine_out_pipe1/1
  Cosine_in_pipe/1 -> Cosine/1
  AddAlpha_stage2/1 -> AddAlpha_stage3/1
  dtc/1 -> Saturation/1
  delayMatch/1 -> reset_old2_controlled/Enable
  delayMatch1/1 -> Delay4_controlled/Enable
  delayMatch2/1 -> Delay5_controlled/Enable
  delayMatch3/1 -> Delay2_controlled/Enable
  delayMatch4/1 -> Delay22_controlled/Enable
  delayMatch7/1 -> Delay7_controlled/Enable
  delayMatch9/1 -> Delay1_controlled/Enable
  delayMatch11/1 -> Delay3_controlled/Enable
  delayMatch14/1 -> Delay10_controlled/Enable
  delayMatch16/1 -> Delay16_controlled/Enable
  stateControl/1 -> delayMatch/1
  stateControl1/1 -> delayMatch1/1
  stateControl2/1 -> delayMatch2/1
  stateControl3/1 -> delayMatch3/1
  stateControl4/1 -> delayMatch4/1
  Add1_out_pipe/1 -> delayMatch5/1, Compare Limit_Low/1, Compare Limit_High/1, Add3/1, Add2/1
  delayMatch10/1 -> Switch_on1/2
  stateControl5/1 -> delayMatch7/1
  stateControl6/1 -> delayMatch9/1
  Saturation/1 -> delayMatch10/1, delayMatch6/1, DelayValue3/1, DelayValid/1, Switch_on3/2, Switch_on4/2, Switch_on2/2
  stateControl7/1 -> delayMatch11/1
  Compare1/1 -> delayMatch13/1
  stateControl8/1 -> delayMatch14/1
  Add4/1 -> delayMatch15/1, Compare1/1, Switch_id/1, Switch_id1/1
  stateControl9/1 -> delayMatch16/1
  out_4_pipe/1 -> delayMatch17/1
  out_7_pipe/1 -> delayMatch18/1
  out_8_pipe/1 -> delayMatch19/1
  out_9_pipe/1 -> delayMatch20/1
  out_10_pipe/1 -> delayMatch21/1
  out_11_pipe/1 -> delayMatch22/1
  out_12_pipe/1 -> delayMatch23/1
  out_13_pipe/1 -> delayMatch24/1
  reset_old_switch1/1 -> reset_old2_controlled/1(in0)
  reset_old2_controlled/1(out0) -> reset_old_switch1/3, Detec_edge/2
  Detec_edge/1 -> 1 for one cycle if edge recognized/1, reset_old_switch1/2
  Delay4_controlled/1(out0) -> Switch_on3/3
  Switch_on3/1 -> Switch_on3_out1/1, Delay4_controlled/1(in0)
  Delay5_controlled/1(out0) -> Switch_on4/3
  Switch_on4/1 -> Switch_on4_out1/1, Delay5_controlled/1(in0)
  Delay2_controlled/1(out0) -> Switch_on2/3
  Switch_on2/1 -> Switch_on2_out1/1, Delay2_controlled/1(in0)
  Delay22_controlled/1(out0) -> Switch_id/4
  Switch_id/1 -> Delay22_controlled/1(in0), delayMatch8/1
  Delay7_controlled/1(out0) -> Switch_on7/3
  Switch_on7/1 -> Delay7_controlled/1(in0), sin1/2
  Delay1_controlled/1(out0) -> Switch_id1/4
  Switch_id1/1 -> Delay1_controlled/1(in0), delayMatch12/1
  Delay3_controlled/1(out0) -> Switch_on1/3
  Switch_on1/1 -> Delay3_controlled/1(in0), cos1/2
  Delay10_controlled/1(out0) -> Switch_idpred1/3
  Switch_idpred1/1 -> Switch_idpred1_out1/1, Delay10_controlled/1(in0)
  Delay16_controlled/1(out0) -> Switch_idpred2/3
  Switch_idpred2/1 -> Switch_idpred2_out1/1, Delay16_controlled/1(in0)

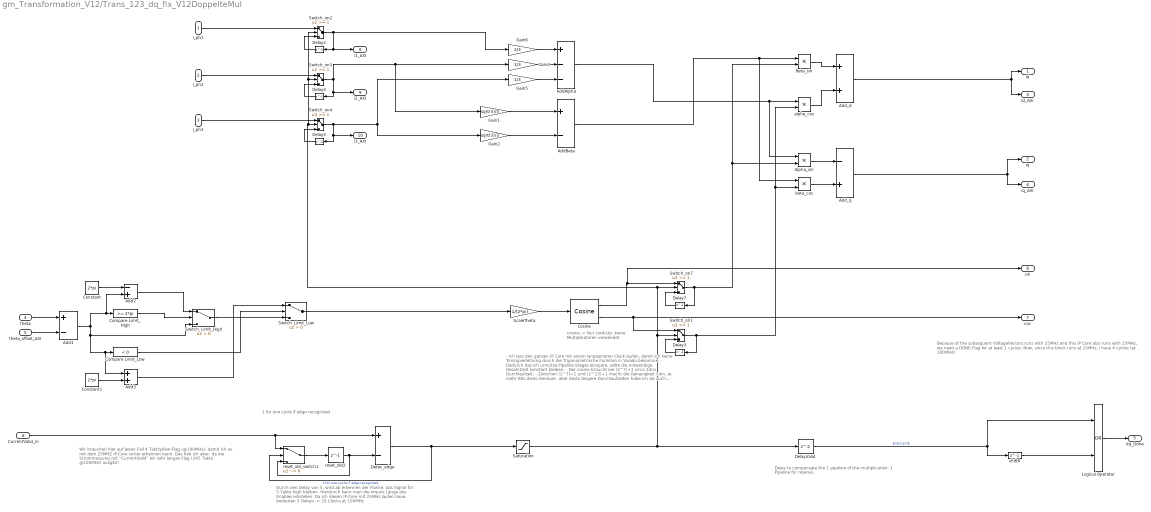
== system gm_Transformation_V12/Trans_123_dq_fix_V12DoppelteMul ==
  note: Because of the subsequent VoltageVectors runs with 25MHz and this
      | IP Core also runs with 25MHz, we need a DONE-Flag for at least 1 cycles.
      | Now, since this block runs at 25MHz, i have 4 cycles (at 100MHz)
  note: Wir brauchen hier auf jeden Fall 4 Taktzyklen-Flag (@100MHz),
      | damit ich es mit dem 25MHZ IP-Core sicher erkennen kann. Das hab
      | ich aber, da die Strommessung mit "CurrentValid" ein sehr langes Flag
      | (345 Takte @100MHz) ausgibt!
  note: 1 for one cycle if edge recognized
  note: Durch den Delay von 5, wird ab erkennen der Flanke,
      |  das Signal für 5 Takte high bleiben.
      | Hierdurch kann man die Impuls Länge des Enables einstellen.
      | Da ich diesen IP-Core mit 25MHz laufen lasse, bedeuten 5 Delays -> 20 Clocks at 100MHz
  note: - Ich lass den ganzen IP Core mit einem langsameren Clock laufen,
      | damit ich keine Timingverletzung durch die Trigonometrische
      | Funktion in Vivado bekomme.
      | - Dadurch das ich unnütze Pipeline Stages einspare, sollte
      | die notwendige Gesamtzeit konstant bleiben.
      | - Der cosine braucht bei (2^7)+1 circa 24ns Durchlaufzeit.
      | - Zwischen (2^7)+1 und (2^13)+1 macht die Genauigkeit Sinn. Je mehr Bits
      | desto Genauer, aber desto längere Durchlaufzeiten habe ich als auch mehr
      | Ressourcen brauche ich. (Habe mich aktuell für (2^9)+1 entschieden.
  note: cosine -> Nur Look-Up,
      | keine Multiplikatoren
      | verwendet
  note: Delay to compensate the 1 pipeline of the multiplication.
      | 1 Pipeline for reserve.
  i_ph1 : Inport
  i_ph2 : Inport  Port=2
  i_ph3 : Inport  Port=3
  theta : Inport  Port=4
  theta_offset_AXI : Inport  Port=5
  CurrentValid_in : Inport  Port=6
  Add1 : Sum  Inputs=+-  OutDataTypeStr=Inherit: Same as accumulator
  Add2 : Sum  Inputs=-+  OutDataTypeStr=Inherit: Same as first input
  Add3 : Sum  OutDataTypeStr=Inherit: Same as first input
  AddAlpha : Sum  Inputs=+--  OutDataTypeStr=Inherit: Same as accumulator  RndMeth=Simplest
  AddBeta : Sum  Inputs=+-  OutDataTypeStr=Inherit: Same as accumulator  RndMeth=Simplest
  Add_d : Sum  OutDataTypeStr=Inherit: Same as accumulator  RndMeth=Simplest
  Add_q : Sum  Inputs=-+  OutDataTypeStr=Inherit: Same as accumulator  RndMeth=Simplest
  Alpha_sin : Product  RndMeth=Simplest  OutDataTypeStr=Inherit: Same as first input
  Beta_sin : Product  RndMeth=Simplest  OutDataTypeStr=Inherit: Same as first input
  Compare Limit_High : simulink/Logic and Bit Operations/Compare To Constant  relop=>=  const=2*pi  OutDataTypeStr=boolean
  Compare Limit_Low : simulink/Logic and Bit Operations/Compare To Constant  relop=<  const=0  OutDataTypeStr=boolean
  Constant : Constant  Value=2*pi  OutDataTypeStr=fixdt(1,24,20)  SampleTime=T_25MHz
  Constant1 : Constant  Value=2*pi  OutDataTypeStr=fixdt(1,24,20)  SampleTime=T_25MHz
  Cosine : simulink/Lookup Tables/Cosine  Formula=sin(2*pi*u) and cos(2*pi*u)  NumDataPoints=(2^9)+1  OutputWordLength=16  InternalRulePriority=Precision
      settings: SourceProductBaseCode=SL
  Delay{2..5,7} (5 alike) : Delay  DelayLength=1
  DelayValid : Delay
  Detec_edge : Sum  Inputs=+-  AccumDataTypeStr=int8  OutDataTypeStr=int8
  Gain1 : Gain  Gain=sqrt(3)/3  OutDataTypeStr=Inherit: Same as input
  Gain2 : Gain  Gain=sqrt(3)/3  OutDataTypeStr=Inherit: Same as input
  Gain4 : Gain  Gain=1/3  OutDataTypeStr=Inherit: Same as input
  Gain5 : Gain  Gain=1/3  OutDataTypeStr=Inherit: Same as input
  Gain6 : Gain  Gain=2/3  OutDataTypeStr=Inherit: Same as input
  Logical Operator : Logic  Operator=OR  AllPortsSameDT=off  OutDataTypeStr=boolean
  Saturation : Saturate  UpperLimit=1  LowerLimit=0  OutMin=[0]  OutMax=[1]  OutDataTypeStr=fixdt(0,1)
  ScaleTheta : Gain  Gain=1/(2*pi)  OutDataTypeStr=Inherit: Same as input
  Switch_Limit_High : Switch  Criteria=u2 > Threshold  OutDataTypeStr=fixdt(1,24,20)  SaturateOnIntegerOverflow=off  InputSameDT=off
  Switch_Limit_Low : Switch  Criteria=u2 > Threshold  OutDataTypeStr=fixdt(1,24,20)  SaturateOnIntegerOverflow=off  InputSameDT=off
  Switch_on1 : Switch  Threshold=1  OutDataTypeStr=fixdt(1,16,14)  SaturateOnIntegerOverflow=off  InputSameDT=off
  Switch_on2 : Switch  Threshold=1  OutDataTypeStr=Inherit: Inherit via back propagation  RndMeth=Simplest  SaturateOnIntegerOverflow=off  InputSameDT=off
  Switch_on3 : Switch  Threshold=1  OutDataTypeStr=Inherit: Inherit via back propagation  RndMeth=Simplest  SaturateOnIntegerOverflow=off  InputSameDT=off
  Switch_on4 : Switch  Threshold=1  OutDataTypeStr=Inherit: Inherit via back propagation  RndMeth=Simplest  SaturateOnIntegerOverflow=off  InputSameDT=off
  Switch_on7 : Switch  Threshold=1  OutDataTypeStr=fixdt(1,16,14)  SaturateOnIntegerOverflow=off  InputSameDT=off
  alpha_cos : Product  RndMeth=Simplest  OutDataTypeStr=Inherit: Same as first input
  beta_cos : Product  RndMeth=Simplest  OutDataTypeStr=Inherit: Same as first input
  reset_old2 : Delay  DelayLength=1
  reset_old_switch1 : Switch  Criteria=u2 ~= 0  SaturateOnIntegerOverflow=off  InputSameDT=off
  shift6 : Delay  DelayLength=1
  id : Outport  VectorParamsAs1DForOutWhenUnconnected=off
  iq : Outport  Port=2  VectorParamsAs1DForOutWhenUnconnected=off
  id_AXI : Outport  Port=3  VectorParamsAs1DForOutWhenUnconnected=off
  iq_AXI : Outport  Port=4  VectorParamsAs1DForOutWhenUnconnected=off
  dq_Done : Outport  Port=5  VectorParamsAs1DForOutWhenUnconnected=off
  sin : Outport  Port=6  VectorParamsAs1DForOutWhenUnconnected=off
  cos : Outport  Port=7  VectorParamsAs1DForOutWhenUnconnected=off
  i1_AXI : Outport  Port=8  VectorParamsAs1DForOutWhenUnconnected=off
  i2_AXI : Outport  Port=9  VectorParamsAs1DForOutWhenUnconnected=off
  i3_AXI : Outport  Port=10  VectorParamsAs1DForOutWhenUnconnected=off
  wires:
  Logical Operator/1 -> dq_Done/1
  shift6/1 -> Logical Operator/2
  DelayValid/1 -> shift6/1, Logical Operator/1  "End_Cycle"
  beta_cos/1 -> Add_q/2
  Alpha_sin/1 -> Add_q/1
  AddBeta/1 -> Beta_sin/1, beta_cos/1
  AddAlpha/1 -> alpha_cos/1, Alpha_sin/1
  alpha_cos/1 -> Add_d/2
  Beta_sin/1 -> Add_d/1
  i_ph3/1 -> Switch_on4/1
  Delay5/1 -> Switch_on4/3
  Switch_on4/1 -> Gain5/1, Gain2/1, Delay5/1, i3_AXI/1
  i_ph2/1 -> Switch_on3/1
  Delay4/1 -> Switch_on3/3
  Switch_on3/1 -> Gain4/1, Gain1/1, Delay4/1, i2_AXI/1
  i_ph1/1 -> Switch_on2/1
  Switch_on2/1 -> Gain6/1, i1_AXI/1, Delay2/1
  Delay2/1 -> Switch_on2/3
  reset_old_switch1/1 -> reset_old2/1
  CurrentValid_in/1 -> Detec_edge/1, reset_old_switch1/1
  reset_old2/1 -> Detec_edge/2, reset_old_switch1/3
  Detec_edge/1 -> reset_old_switch1/2, Saturation/1  "1 for one cycle if edge recognized"
  Gain6/1 -> AddAlpha/1
  Gain5/1 -> AddAlpha/3
  Gain4/1 -> AddAlpha/2
  Switch_Limit_Low/1 -> ScaleTheta/1
  Switch_on1/1 -> alpha_cos/2, beta_cos/2, Delay3/1
  Cosine/1 -> Switch_on7/1, sin/1
  Switch_on7/1 -> Alpha_sin/2, Beta_sin/2, Delay7/1
  Cosine/2 -> cos/1, Switch_on1/1
  ScaleTheta/1 -> Cosine/1
  Delay7/1 -> Switch_on7/3
  Delay3/1 -> Switch_on1/3
  Saturation/1 -> Switch_on7/2, Switch_on4/2, Switch_on3/2, Switch_on2/2, Switch_on1/2, DelayValid/1
  Add_d/1 -> id_AXI/1, id/1
  Add_q/1 -> iq_AXI/1, iq/1
  Add3/1 -> Switch_Limit_Low/1
  Constant1/1 -> Add3/2
  Add2/1 -> Switch_Limit_High/1
  Constant/1 -> Add2/1
  Compare Limit_Low/1 -> Switch_Limit_Low/2
  Compare Limit_High/1 -> Switch_Limit_High/2
  Switch_Limit_High/1 -> Switch_Limit_Low/3
  theta_offset_AXI/1 -> Add1/2
  Add1/1 -> Compare Limit_High/1, Add2/2, Compare Limit_Low/1, Add3/1, Switch_Limit_High/3
  theta/1 -> Add1/1
  Gain2/1 -> AddBeta/2
  Gain1/1 -> AddBeta/1

== system gm_Transformation_V12/Trans_123_dq_fix_V3 ==
  i_ph1 : Inport
  i_ph3 : Inport  Port=2
  theta : Inport  Port=3
  Add : Sum
  Gain1 : Gain  Gain=1/sqrt(3)  OutDataTypeStr=Inherit: Same as input
  Gain2 : Gain  Gain=2/sqrt(3)  OutDataTypeStr=Inherit: Same as input
  dq_transformation : MATLAB Function  TreatAsAtomicUnit=on
  id : Outport  VectorParamsAs1DForOutWhenUnconnected=off
  iq : Outport  Port=2  VectorParamsAs1DForOutWhenUnconnected=off
  wires:
  theta/1 -> dq_transformation/3(theta)
  i_ph3/1 -> Gain2/1
  dq_transformation/1(d) -> id/1
  dq_transformation/2(q) -> iq/1
  Gain2/1 -> Add/2
  Gain1/1 -> Add/1
  Add/1 -> dq_transformation/2(b)
  i_ph1/1 -> Gain1/1, dq_transformation/1(a)

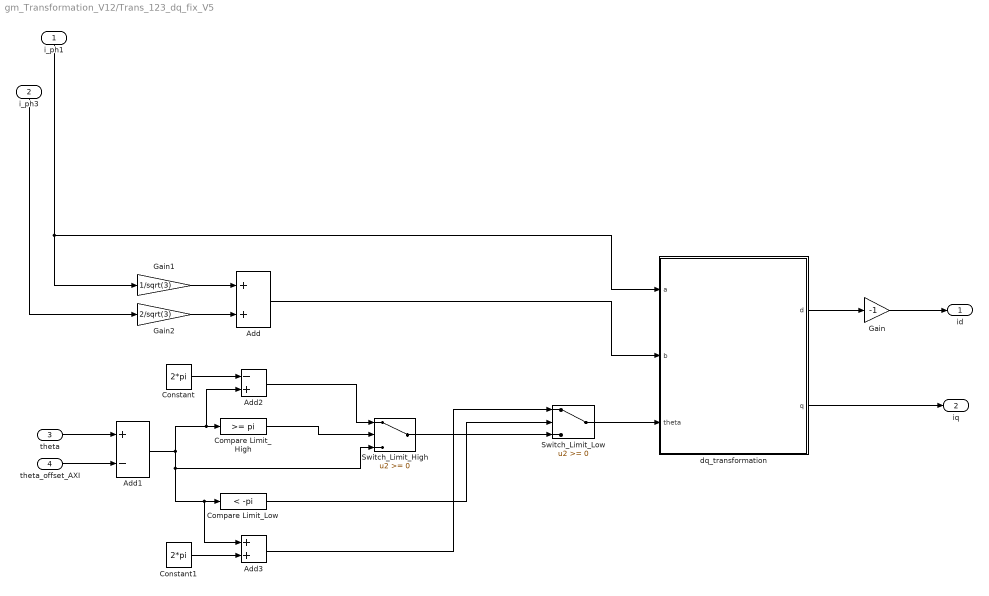
== system gm_Transformation_V12/Trans_123_dq_fix_V5 ==
  i_ph1 : Inport
  i_ph3 : Inport  Port=2
  theta : Inport  Port=3
  theta_offset_AXI : Inport  Port=4
  Add : Sum
  Add1 : Sum  Inputs=+-  OutDataTypeStr=Inherit: Same as accumulator
  Add2 : Sum  Inputs=-+  OutDataTypeStr=Inherit: Same as first input
  Add3 : Sum  OutDataTypeStr=Inherit: Same as first input
  Compare Limit_High : simulink/Logic and Bit Operations/Compare To Constant  relop=>=  const=pi  OutDataTypeStr=boolean
  Compare Limit_Low : simulink/Logic and Bit Operations/Compare To Constant  relop=<  const=-pi  OutDataTypeStr=boolean
  Constant : Constant  Value=2*pi  OutDataTypeStr=fixdt(1,24,20)  SampleTime=-1
  Constant1 : Constant  Value=2*pi  OutDataTypeStr=fixdt(1,24,20)  SampleTime=-1
  Gain : Gain  Gain=-1  OutDataTypeStr=Inherit: Same as input
  Gain1 : Gain  Gain=1/sqrt(3)  OutDataTypeStr=Inherit: Same as input
  Gain2 : Gain  Gain=2/sqrt(3)  OutDataTypeStr=Inherit: Same as input
  Switch_Limit_High : Switch  OutDataTypeStr=fixdt(1,24,20)  SaturateOnIntegerOverflow=off  InputSameDT=off
  Switch_Limit_Low : Switch  OutDataTypeStr=fixdt(1,24,20)  SaturateOnIntegerOverflow=off  InputSameDT=off
  dq_transformation : MATLAB Function  TreatAsAtomicUnit=on
  id : Outport  VectorParamsAs1DForOutWhenUnconnected=off
  iq : Outport  Port=2  VectorParamsAs1DForOutWhenUnconnected=off
  wires:
  Gain/1 -> id/1
  Add3/1 -> Switch_Limit_Low/1
  Constant1/1 -> Add3/2
  Add2/1 -> Switch_Limit_High/1
  Constant/1 -> Add2/1
  Compare Limit_Low/1 -> Switch_Limit_Low/2
  Compare Limit_High/1 -> Switch_Limit_High/2
  Switch_Limit_High/1 -> Switch_Limit_Low/3
  Switch_Limit_Low/1 -> dq_transformation/3(theta)
  theta_offset_AXI/1 -> Add1/2
  Add1/1 -> Compare Limit_High/1, Add2/2, Compare Limit_Low/1, Add3/1, Switch_Limit_High/3
  theta/1 -> Add1/1
  i_ph3/1 -> Gain2/1
  dq_transformation/1(d) -> Gain/1
  dq_transformation/2(q) -> iq/1
  Gain2/1 -> Add/2
  Gain1/1 -> Add/1
  Add/1 -> dq_transformation/2(b)
  i_ph1/1 -> Gain1/1, dq_transformation/1(a)

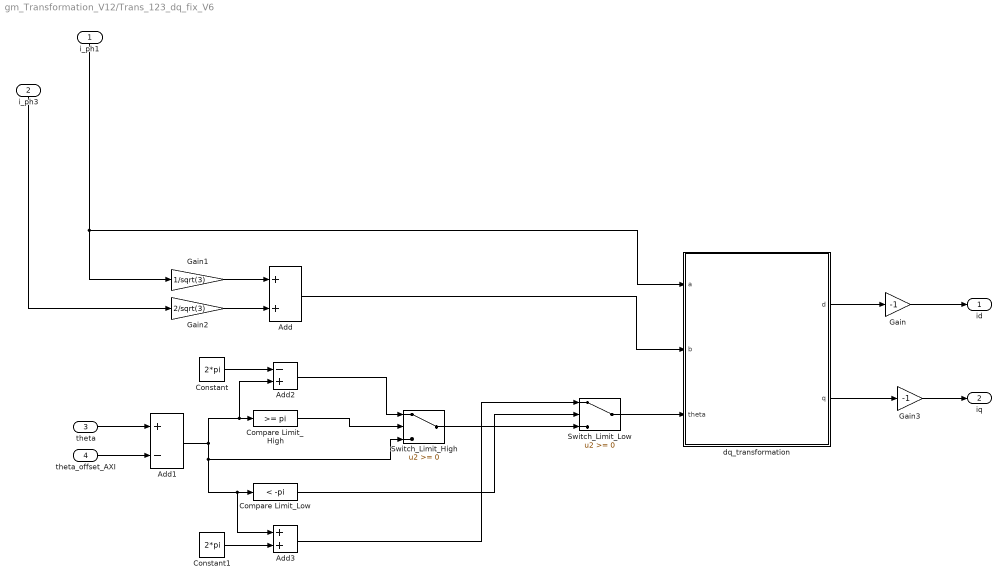
== system gm_Transformation_V12/Trans_123_dq_fix_V6 ==
  i_ph1 : Inport
  i_ph3 : Inport  Port=2
  theta : Inport  Port=3
  theta_offset_AXI : Inport  Port=4
  Add : Sum
  Add1 : Sum  Inputs=+-  OutDataTypeStr=Inherit: Same as accumulator
  Add2 : Sum  Inputs=-+  OutDataTypeStr=Inherit: Same as first input
  Add3 : Sum  OutDataTypeStr=Inherit: Same as first input
  Compare Limit_High : simulink/Logic and Bit Operations/Compare To Constant  relop=>=  const=pi  OutDataTypeStr=boolean
  Compare Limit_Low : simulink/Logic and Bit Operations/Compare To Constant  relop=<  const=-pi  OutDataTypeStr=boolean
  Constant : Constant  Value=2*pi  OutDataTypeStr=fixdt(1,24,20)  SampleTime=-1
  Constant1 : Constant  Value=2*pi  OutDataTypeStr=fixdt(1,24,20)  SampleTime=-1
  Gain : Gain  Gain=-1  OutDataTypeStr=fixdt(1,18,11)
  Gain1 : Gain  Gain=1/sqrt(3)  OutDataTypeStr=Inherit: Same as input
  Gain2 : Gain  Gain=2/sqrt(3)  OutDataTypeStr=Inherit: Same as input
  Gain3 : Gain  Gain=-1  OutDataTypeStr=fixdt(1,18,11)
  Switch_Limit_High : Switch  OutDataTypeStr=fixdt(1,24,20)  SaturateOnIntegerOverflow=off  InputSameDT=off
  Switch_Limit_Low : Switch  OutDataTypeStr=fixdt(1,24,20)  SaturateOnIntegerOverflow=off  InputSameDT=off
  dq_transformation : MATLAB Function  TreatAsAtomicUnit=on
  id : Outport  VectorParamsAs1DForOutWhenUnconnected=off
  iq : Outport  Port=2  VectorParamsAs1DForOutWhenUnconnected=off
  wires:
  Gain3/1 -> iq/1
  Gain/1 -> id/1
  Add3/1 -> Switch_Limit_Low/1
  Constant1/1 -> Add3/2
  Add2/1 -> Switch_Limit_High/1
  Constant/1 -> Add2/1
  Compare Limit_Low/1 -> Switch_Limit_Low/2
  Compare Limit_High/1 -> Switch_Limit_High/2
  Switch_Limit_High/1 -> Switch_Limit_Low/3
  Switch_Limit_Low/1 -> dq_transformation/3(theta)
  theta_offset_AXI/1 -> Add1/2
  Add1/1 -> Compare Limit_High/1, Add2/2, Compare Limit_Low/1, Add3/1, Switch_Limit_High/3
  theta/1 -> Add1/1
  i_ph3/1 -> Gain2/1
  dq_transformation/1(d) -> Gain/1
  dq_transformation/2(q) -> Gain3/1
  Gain2/1 -> Add/2
  Gain1/1 -> Add/1
  Add/1 -> dq_transformation/2(b)
  i_ph1/1 -> Gain1/1, dq_transformation/1(a)

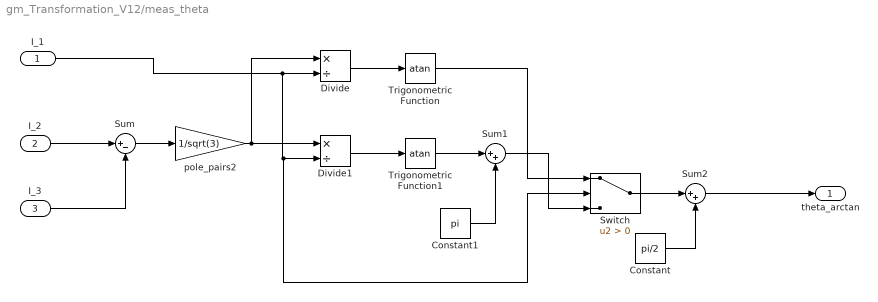
== system gm_Transformation_V12/meas_theta ==
  I_1 : Inport
  I_2 : Inport  Port=2
  I_3 : Inport  Port=3
  Constant : Constant  Value=pi/2
  Constant1 : Constant  Value=pi
  Divide : Product  Inputs=*/
  Divide1 : Product  Inputs=*/
  Sum : Sum  Inputs=|+-
  Sum1 : Sum  Inputs=|++
  Sum2 : Sum  Inputs=|++
  Switch : Switch  Criteria=u2 > Threshold  SaturateOnIntegerOverflow=off  InputSameDT=off
  Trigonometric Function : Trigonometry  Operator=atan
  Trigonometric Function1 : Trigonometry  Operator=atan
  pole_pairs2 : Gain  Gain=1/sqrt(3)
  theta_arctan : Outport  VectorParamsAs1DForOutWhenUnconnected=off
  wires:
  Sum2/1 -> theta_arctan/1
  Constant1/1 -> Sum1/2
  Constant/1 -> Sum2/2
  Switch/1 -> Sum2/1
  Trigonometric Function/1 -> Switch/1
  Sum1/1 -> Switch/3
  I_1/1 -> Divide/2, Divide1/2, Switch/2
  I_2/1 -> Sum/1
  I_3/1 -> Sum/2
  Sum/1 -> pole_pairs2/1
  pole_pairs2/1 -> Divide1/1, Divide/1
  Trigonometric Function1/1 -> Sum1/1
  Divide1/1 -> Trigonometric Function1/1
  Divide/1 -> Trigonometric Function/1

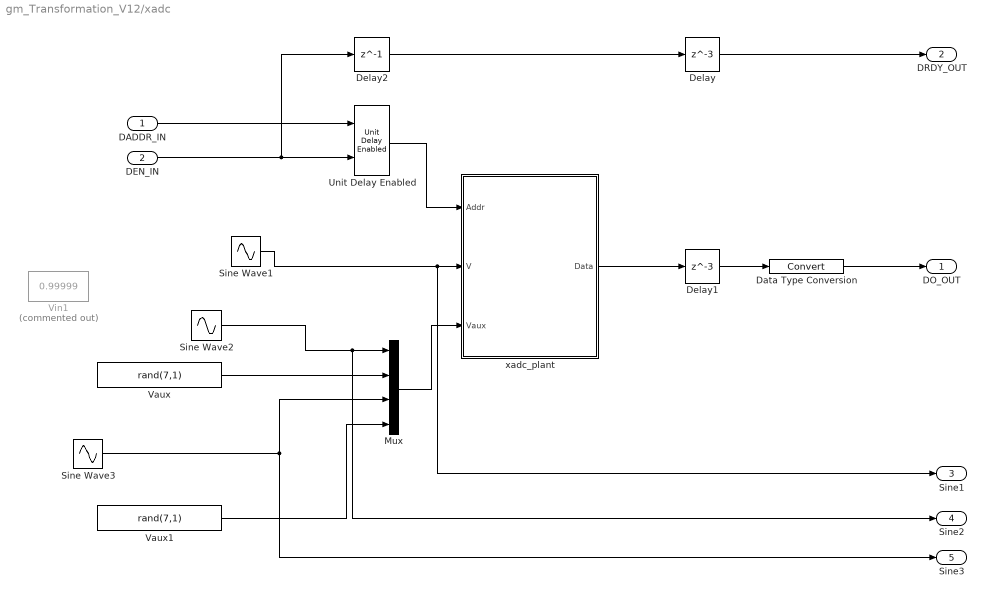
== system gm_Transformation_V12/xadc ==
  DADDR_IN : Inport  OutDataTypeStr=fixdt(0,7,0)
  DEN_IN : Inport  Port=2  OutDataTypeStr=boolean
  Data Type Conversion : DataTypeConversion  SaturateOnIntegerOverflow=off  RndMeth=Floor
  Delay : Delay  DelayLength=3
  Delay1 : Delay  DelayLength=3
  Delay2 : Delay  DelayLength=1
  Mux : Mux
  Sine Wave1 : Sin  Amplitude=0.49  Bias=0.5  Frequency=50  SampleTime=T_mech
  Sine Wave2 : Sin  Amplitude=0.49  Bias=0.5  Frequency=50  Phase=-2*pi/3  SampleTime=T_mech
  Sine Wave3 : Sin  Amplitude=0.49  Bias=0.5  Frequency=50  Phase=2*pi/3  SampleTime=T_mech
  Unit Delay Enabled : simulink_need_slupdate/Unit Delay Enabled  vinit=0.0  tsamp=-1
      settings: SourceProductBaseCode=SL
  Vaux : Constant  Value=rand(7,1)  SampleTime=-1
  Vaux1 : Constant  Value=rand(7,1)  SampleTime=-1
  Vin1 : Constant  Commented=on  Value=0.99999  SampleTime=-1
  xadc_plant : Subsystem
  DO_OUT : Outport  OutDataTypeStr=fixdt(0,16,0)  VectorParamsAs1DForOutWhenUnconnected=off
  DRDY_OUT : Outport  Port=2  OutDataTypeStr=boolean  VectorParamsAs1DForOutWhenUnconnected=off
  Sine1 : Outport  Port=3  VectorParamsAs1DForOutWhenUnconnected=off
  Sine2 : Outport  Port=4  VectorParamsAs1DForOutWhenUnconnected=off
  Sine3 : Outport  Port=5  VectorParamsAs1DForOutWhenUnconnected=off
  wires:
  Mux/1 -> xadc_plant/3(Vaux)
  Sine Wave2/1 -> Mux/1, Sine2/1
  Sine Wave3/1 -> Sine3/1, Mux/3
  Vaux1/1 -> Mux/4
  Vaux/1 -> Mux/2
  Sine Wave1/1 -> xadc_plant/2(V), Sine1/1
  Unit Delay Enabled/1 -> xadc_plant/1(Addr)
  xadc_plant/1(Data) -> Delay1/1
  Delay2/1 -> Delay/1
  Delay1/1 -> Data Type Conversion/1
  Delay/1 -> DRDY_OUT/1
  Data Type Conversion/1 -> DO_OUT/1
  DADDR_IN/1 -> Unit Delay Enabled/1
  DEN_IN/1 -> Unit Delay Enabled/2, Delay2/1
